simulink model "calcul_Mz_PID"  (R2024b)
settings: Solver=FixedStepAuto  StartTime=0.0  StopTime=10.0  FixedStep=Ts  RelTol=1e-3
undefined symbols (not defined in the file): Cf, Cr, Ki, Kp, lf, lr, m, TV
settings Model: Creator=marti  LastModifiedBy=Filip

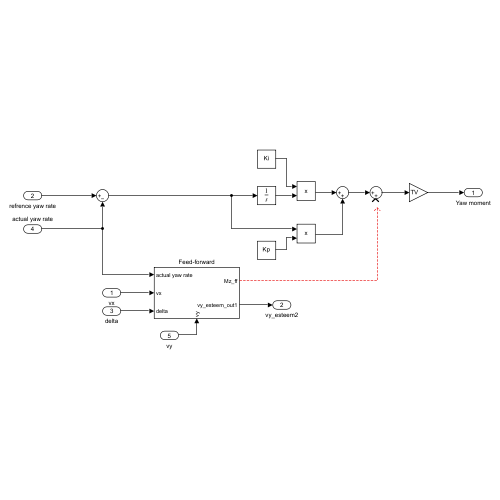
[thumbnail: Simulink's stored preview of the top-level diagram]
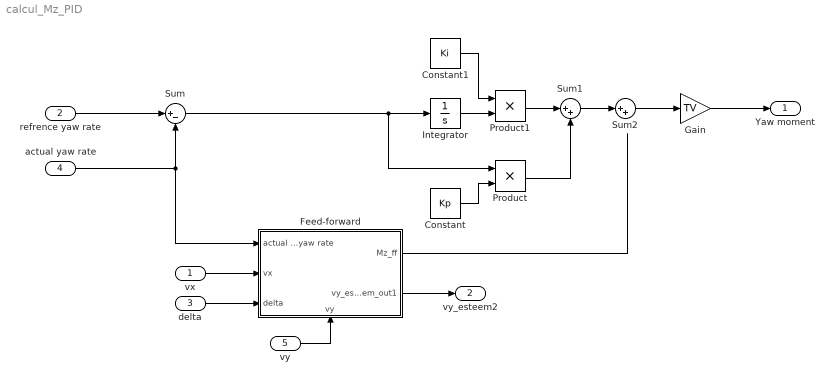
== system calcul_Mz_PID ==
  vx : Inport
  refrence yaw rate : Inport  Port=2
  delta : Inport  Port=3
  actual yaw rate : Inport  Port=4
  vy : Inport  Port=5
  Constant : Constant  Value=Kp
  Constant1 : Constant  Value=Ki
  Feed-forward : Subsystem
      settings: PortSchema="{\"entries\":[{\"content\":{\"sides\":[{\"content\":{\"connectorIds\":[\"In1\",\"In2\",\"In3\"]},\"type\":\"ConnectorPlacement.EquallySpacedRectSide\",\"uuid\":\"af8368cf-4f84-4250-9673-79f62898b3cc\"},{\"content\":{\"connectorIds\":[\"Out1\",\"Out2\"],\"side\":\"RIGHT\"},\"type\":\"ConnectorPlacement.EquallySpacedRectSide\",\"uuid\":\"09f02962-5c7c-4455-ad81-befc240d6e55\"},{\"content\":{\"side\":\"TOP\"},\"type\":\"ConnectorPlacement.EquallySpacedRectSide\",\"uuid\":\"7a5fb401-319c-4a88-af01-2dc8b8cc2b6a\"},{\"content\":{\"connectorIds\":[\"In4\"],\"side\":\"BOTTOM\"},\"type\":\"ConnectorPlacement.EquallySpacedRectSide\",\"uuid\":\"65b1ac5c-7626-4bf0-b657-0a59cfe23dc9\"}]},\"type\":\"ConnectorPlacement.EquallySpacedConnector\",\"uuid\":\"62a1c25a-eba9-43b8-a069-759f180a4ce0\"}],\"packageUris\":[\"http://schema.mathworks.com/mf0/Connector/R2020b\"],\"version\":\"1.0\"}"
  Gain : Gain  Gain=TV
  Integrator : Integrator
  Product : Product
  Product1 : Product
  Sum : Sum  Inputs=|+-
  Sum1 : Sum  Inputs=|++
  Sum2 : Sum  Inputs=|++
  Yaw moment : Outport
  vy_esteem2 : Outport  Port=2
  wires:
  refrence yaw rate/1 -> Sum/1
  Sum1/1 -> Sum2/1
  actual yaw rate/1 -> Feed-forward/1(actual yaw rate), Sum/2
  Sum/1 -> Product/1, Integrator/1
  Constant/1 -> Product/2
  Integrator/1 -> Product1/2
  Constant1/1 -> Product1/1
  Product1/1 -> Sum1/1
  Product/1 -> Sum1/2
  delta/1 -> Feed-forward/3(delta)
  vx/1 -> Feed-forward/2(vx)
  Feed-forward/2(vy_esteem_out1) -> vy_esteem2/1
  Sum2/1 -> Gain/1
  Feed-forward/1(Mz_ff) -> ?
  vy/1 -> Feed-forward/4(vy)
  Gain/1 -> Yaw moment/1

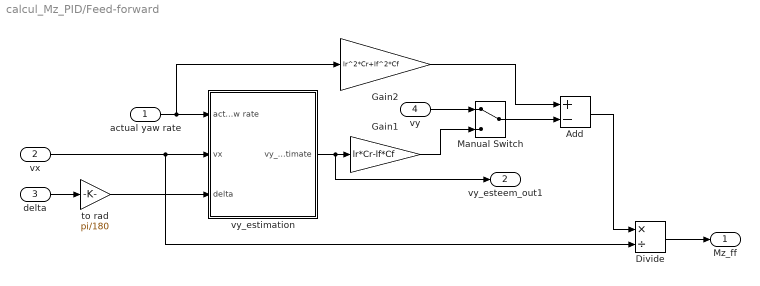
== system calcul_Mz_PID/Feed-forward ==
  actual yaw rate : Inport
  vx : Inport  Port=2
  delta : Inport  Port=3
  vy : Inport  Port=4
  Add : Sum  Inputs=+-
  Divide : Product  Inputs=*/
  Gain1 : Gain  Gain=lr*Cr-lf*Cf
  Gain2 : Gain  Gain=lr^2*Cr+lf^2*Cf
  Manual Switch : ManualSwitch
  to rad : Gain  Gain=pi/180
  vy_estimation : Subsystem
  Mz_ff : Outport
  vy_esteem_out1 : Outport  Port=2
  wires:
  vx/1 -> Divide/2, vy_estimation/2(vx)
  Gain2/1 -> Add/1
  delta/1 -> to rad/1
  vy_estimation/1(vy_estimate) -> vy_esteem_out1/1, Gain1/1
  Add/1 -> Divide/1
  Gain1/1 -> Manual Switch/2
  Divide/1 -> Mz_ff/1
  actual yaw rate/1 -> Gain2/1, vy_estimation/1(actual yaw rate)
  Manual Switch/1 -> Add/2
  vy/1 -> Manual Switch/1
  to rad/1 -> vy_estimation/3(delta)

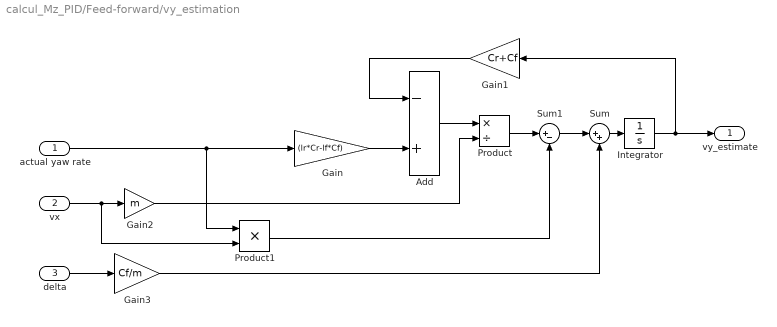
== system calcul_Mz_PID/Feed-forward/vy_estimation ==
  actual yaw rate : Inport
  vx : Inport  Port=2
  delta : Inport  Port=3
  Add : Sum  Inputs=-+
  Gain : Gain  Gain=(lr*Cr-lf*Cf)
  Gain1 : Gain  Gain=Cr+Cf
  Gain2 : Gain  Gain=m
  Gain3 : Gain  Gain=Cf/m
  Integrator : Integrator
  Product : Product  Inputs=*/
  Product1 : Product
  Sum : Sum  Inputs=|++
  Sum1 : Sum  Inputs=|+-
  vy_estimate : Outport
  wires:
  Integrator/1 -> vy_estimate/1, Gain1/1
  Gain/1 -> Add/2
  delta/1 -> Gain3/1
  Gain1/1 -> Add/1
  Add/1 -> Product/1
  Gain2/1 -> Product/2
  Product/1 -> Sum1/1
  vx/1 -> Product1/2, Gain2/1
  actual yaw rate/1 -> Product1/1, Gain/1
  Sum/1 -> Integrator/1
  Gain3/1 -> Sum/2
  Sum1/1 -> Sum/1
  Product1/1 -> Sum1/2
